simulink library "Springs_Axle2"  (R2026a)
settings: Solver=VariableStepAuto
undefined symbols (not defined in the file): Vehicle
libraries: sm_car_lib x1, Springs_Axle2_Decoupled x1, Springs_Axle2_Independent x1, Springs_Axle2_Interconnected x1, Springs_Axle2_Linear x1, Springs_Axle2_None x1
Description:
  | Component of Simscape Vehicle Templates Library
  | 
  | Copyright 2018-2026 The MathWorks, Inc.
settings Model: Creator=smiller  LastModifiedBy=smiller

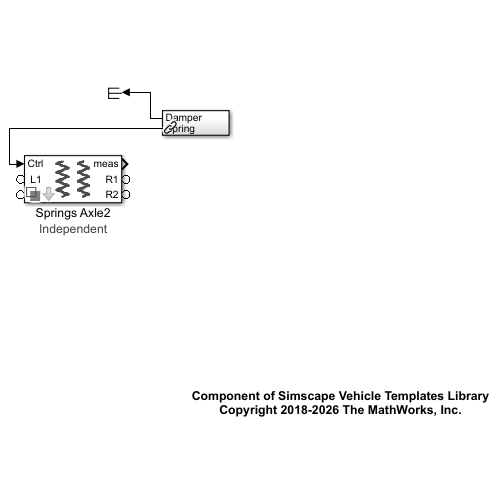
[thumbnail: Simulink's stored preview of the top-level diagram]
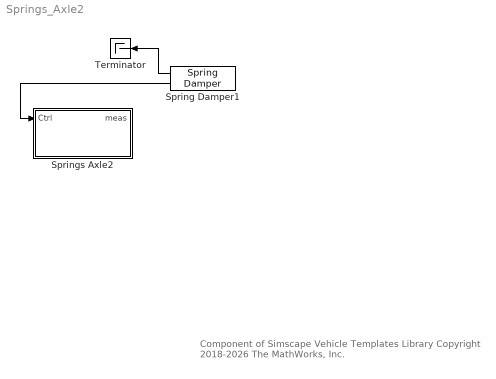
== system Springs_Axle2 ==
  note: Component of Simscape Vehicle Templates Library
      | Copyright 2018-2026 The MathWorks, Inc.
  Spring Damper1 : sm_car_lib/Inputs/Control Bus/Spring Damper  SystemSampleTime=-1  VariantActivationTime=update diagram  EmptyChoice=off  PassThrough=off  PassThroughVariantControl=(default)  EmptyChoiceVariantControl=(default)  AllowFlexibleInterface=on  Latency=0  AutoFrameSizeCalculation=off
  Springs Axle2 : Subsystem  Variant=on  VariantControlMode=label  VariantControl=Variant1  LabelModeActiveChoice=Independent  mask(Variants for Springs){Spring=Vehicle.Chassis.Spring, VariantLabel=Vehicle.Chassis.Spring.class.Value, InitTriggerDropdown=1}
      mask prompts: Spring "Spring Parameters"; VariantLabel "Variant Label"; InitTriggerDropdown "Initialization Trigger Dropdown"
      mask help: Select option and provide parameters for left and right springs on two axles. Option is chosen by string provided in Variant Label. The parameters for the selected option is contained in Springs data structure.
      mask init:
      | curblk = gcb;
      | 
      | % Set variant for this block 
      | set_param(curblk,'LabelModeActiveChoice',VariantLabel);
      | 
      | % Trigger Mask Initialization for 
      | % variant subsystems below this level
      | sm_car_lib_maskInitTrigger(curblk);
      settings: AttributesFormatString=%<ActiveVariant>
      mask TypeOptions InitTriggerDropdown: 0 | 1
      mask Display:
      | if(strcmp(get_param(gcb,'LabelModeActiveChoice'),'None'))
      |     disp(' ');
      | else
      |     image('sm_car_vehicle_chassis_spring_IMAGE.png');
      | end
  Terminator : Terminator
  wires:
  Spring Damper1/1 -> Terminator/1
  Spring Damper1/2 -> Springs Axle2/1("Ctrl ")

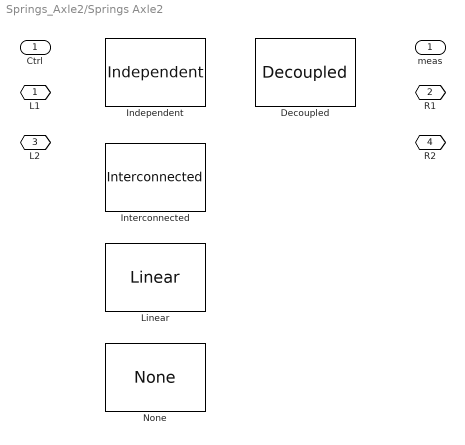
== system Springs_Axle2/Springs Axle2 ==
  "Ctrl " : Inport
  Decoupled : Springs_Axle2_Decoupled/Decoupled  VariantControl=Decoupled  InitTriggerDropdown=1
  Independent : Springs_Axle2_Independent/Independent  VariantControl=Independent  InitTriggerDropdown=1
  Interconnected : Springs_Axle2_Interconnected/Interconnected  VariantControl=Interconnected  InitTriggerDropdown=0
  Linear : Springs_Axle2_Linear/Linear  SystemSampleTime=-1  VariantControl=Linear  VariantActivationTime=update diagram  EmptyChoice=off  PassThrough=off  PassThroughVariantControl=(default)  EmptyChoiceVariantControl=(default)  AllowFlexibleInterface=on  Latency=0  AutoFrameSizeCalculation=off
  None : Springs_Axle2_None/None  VariantControl=None  InitTriggerDropdown=1
  " L1" : PMIOPort  Side=Left
  R1 : PMIOPort  Port=2  Side=Right
  " L2" : PMIOPort  Port=3  Side=Left
  R2 : PMIOPort  Port=4  Side=Right
  " meas" : Outport  VectorParamsAs1DForOutWhenUnconnected=off
